simulink model "sltestRollRefTestExample"  (R2019a)
settings: Solver=FixedStepDiscrete  StartTime=0.0  StopTime=50  RelTol=1e-3
libraries: simulink x1, simulink_need_slupdate x1
settings Model: Creator=The MathWorks, Inc.  LastModifiedBy=sjayagop
settings DataIOCC: ReturnWorkspaceOutputs=off
settings DebuggingCC: PregeneratedLibrarySubsystemCodeDiagnostic=none  SFUnusedDataAndEventsDiag=none  ArithmeticOperatorsInVariantConditions=warning
settings SFSimCC: SimUseLocalCustomCode=off
settings RTWCC: RTWUseLocalCustomCode=off
settings CodeAppCC: StateflowObjectComments=on
settings ConfigComp: CovMetricSettings=dswe

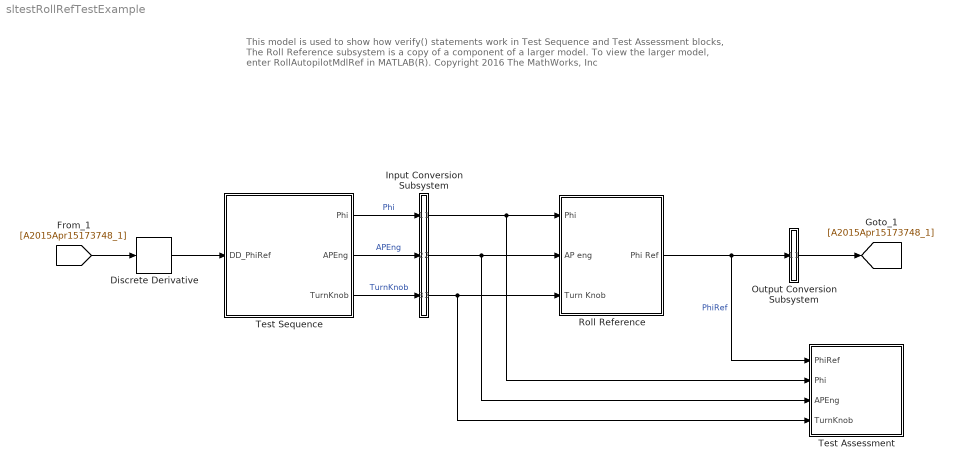
== system sltestRollRefTestExample ==
  note: This model is used to show how verify() statements work in Test Sequence and Test Assessment blocks,
      | The Roll Reference subsystem is a copy of a component of a larger model.
      | To view the larger model, enter RollAutopilotMdlRef in MATLAB(R).
      |
      | Copyright 2016 The MathWorks, Inc
  Discrete Derivative : simulink/Discrete/Discrete Derivative  gainval=1.0  ICPrevScaledInput=0.0  OutMin=[]  OutMax=[]  OutDataType=fixdt(1, 16)  OutScaling=2^-10  DoSatur=off
  Input Conversion Subsystem : Subsystem  Tag=_input_conv_ss_
  Output Conversion Subsystem : Subsystem  Tag=_output_conv_ss_
  Roll Reference : Subsystem  RequirementInfo={'other' 'RollAutopilotRequirements.txt' '?1.3 Roll Hold Reference' 'true' '1.3 Roll Hold Reference' '' } %GIDa_a6fe2b3a_fc40_48ad_979d_ac7ba21092bc  TreatAsAtomicUnit=on
      settings: RTWSystemCode=Inline
  Test Assessment : Test Sequence  TreatAsAtomicUnit=on
  Test Sequence : Test Sequence  RequirementInfo={'linktype_rmi_testmgr' 'AutopilotTestFile.mldatx' '635fd623-8d91-4a63-9a87-5e8aa5687fc0' 'true' 'Test Case Requirement 1.3 Test in AutopilotTestFile' '' } %GIDa_03a19a86_3761_446b_82d3_438f47eaa67c  TreatAsAtomicUnit=on
  wires:
  [A2015Apr15173748_1] -> Discrete Derivative/1
  Test Sequence/1(Phi) -> Input Conversion Subsystem/1(In_1)  "Phi"
  Test Sequence/2(APEng) -> Input Conversion Subsystem/2(In_2)  "APEng"
  Test Sequence/3(TurnKnob) -> Input Conversion Subsystem/3(In_3)  "TurnKnob"
  Input Conversion Subsystem/1(Out_1) -> Roll Reference/1(Phi), Test Assessment/2(Phi)
  Input Conversion Subsystem/2(Out_2) -> Roll Reference/2(AP eng), Test Assessment/3(APEng)
  Input Conversion Subsystem/3(Out_3) -> Roll Reference/3(Turn Knob), Test Assessment/4(TurnKnob)
  Roll Reference/1(Phi Ref) -> Test Assessment/1(PhiRef), Output Conversion Subsystem/1(In_1)  "PhiRef"
  Output Conversion Subsystem/1(Out_1) -> [A2015Apr15173748_1]
  Discrete Derivative/1 -> Test Sequence/1(DD_PhiRef)

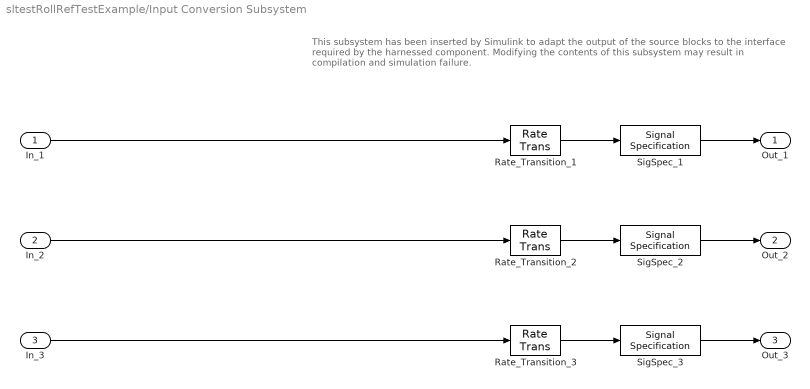
== system sltestRollRefTestExample/Input Conversion Subsystem ==
  note: This subsystem has been inserted by Simulink to adapt the output of the source blocks to the interface required by the harnessed component.
      |  Modifying the contents of this subsystem may result in compilation and simulation failure.
  In_1 : Inport
  In_2 : Inport  Port=2
  In_3 : Inport  Port=3
  Rate_Transition_1 : RateTransition  OutPortSampleTime=0.025
  Rate_Transition_2 : RateTransition  OutPortSampleTime=0.025
  Rate_Transition_3 : RateTransition  OutPortSampleTime=0.025
  SigSpec_1 : SignalSpecification  OutDataTypeStr=double  Dimensions=[1]  SampleTime=0.025
  SigSpec_2 : SignalSpecification  OutDataTypeStr=boolean  Dimensions=[1]  SampleTime=0.025
  SigSpec_3 : SignalSpecification  OutDataTypeStr=double  Dimensions=[1]  SampleTime=0.025
  Out_1 : Outport
  Out_2 : Outport  Port=2
  Out_3 : Outport  Port=3
  wires:
  In_1/1 -> Rate_Transition_1/1
  In_2/1 -> Rate_Transition_2/1
  In_3/1 -> Rate_Transition_3/1
  Rate_Transition_1/1 -> SigSpec_1/1
  Rate_Transition_2/1 -> SigSpec_2/1
  Rate_Transition_3/1 -> SigSpec_3/1
  SigSpec_1/1 -> Out_1/1
  SigSpec_2/1 -> Out_2/1
  SigSpec_3/1 -> Out_3/1

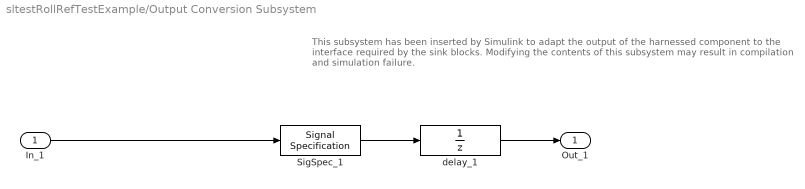
== system sltestRollRefTestExample/Output Conversion Subsystem ==
  note: This subsystem has been inserted by Simulink to adapt the output of the harnessed component to the interface required by the sink blocks.
      |  Modifying the contents of this subsystem may result in compilation and simulation failure.
  In_1 : Inport
  SigSpec_1 : SignalSpecification  OutDataTypeStr=double  Dimensions=[1]  SampleTime=0.025
  delay_1 : UnitDelay  SampleTime=-1  HasFrameUpgradeWarning=on
  Out_1 : Outport
  wires:
  delay_1/1 -> Out_1/1
  SigSpec_1/1 -> delay_1/1
  In_1/1 -> SigSpec_1/1

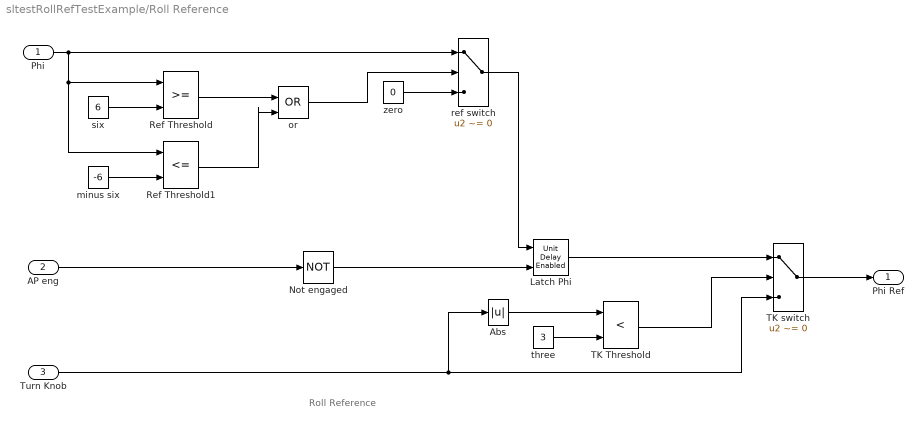
== system sltestRollRefTestExample/Roll Reference ==
  note: Roll Reference
  Phi : Inport  RequirementInfo={'other' 'RollAutopilotRequirements.txt' '?1.3 Roll Hold Reference' 'true' '1.3 Roll Hold Reference' '' } %GIDa_191cb6f5_9fbe_4640_9b65_3b39d8becb52
  AP eng : Inport  RequirementInfo={'other' 'RollAutopilotRequirements.txt' '?1.3 Roll Hold Reference' 'true' '1.3 Roll Hold Reference' '' } %GIDa_123acc0c_25f5_45e7_ac3a_1f2518b48f3f  Port=2
  Turn Knob : Inport  RequirementInfo={'other' 'RollAutopilotRequirements.txt' '?1.3 Roll Hold Reference' 'true' '1.3 Roll Hold Reference' '' } %GIDa_b6599344_476f_4c9f_9990_af58eba30b01  Port=3
  Abs : Abs  RequirementInfo={'other' 'RollAutopilotRequirements.txt' '?1.3 Roll Hold Reference' 'true' '1.3 Roll Hold Reference' '' } %GIDa_3ae1946e_a95c_4cb7_ad5c_447f76069b53
  Latch Phi : simulink_need_slupdate/Unit Delay Enabled  RequirementInfo={'other' 'RollAutopilotRequirements.txt' '?1.3 Roll Hold Reference' 'true' '1.3 Roll Hold Reference' '' } %GIDa_4d4d235f_0389_4d32_a678_f192d33a24f1  vinit=0.0  tsamp=1/40
      settings: SourceProductName=Simulink  SourceProductBaseCode=SL
  Not engaged : Logic  RequirementInfo={'other' 'RollAutopilotRequirements.txt' '?1.3 Roll Hold Reference' 'true' '1.3 Roll Hold Reference' '' } %GIDa_f773b49d_367f_448f_8750_15955fcab6a4  Operator=NOT  IconShape=distinctive  AllPortsSameDT=off  OutDataTypeStr=boolean
  Ref Threshold : RelationalOperator  RequirementInfo={'other' 'RollAutopilotRequirements.txt' '?1.3 Roll Hold Reference' 'true' '1.3 Roll Hold Reference' '' } %GIDa_215460f1_09d0_4074_847e_2cd07dedce05  OutDataTypeStr=boolean  RndMeth=Nearest  InputSameDT=on
  Ref Threshold1 : RelationalOperator  RequirementInfo={'other' 'RollAutopilotRequirements.txt' '?1.3 Roll Hold Reference' 'true' '1.3 Roll Hold Reference' '' } %GIDa_bbe88d87_da81_4bf6_a41e_c7cf823cfa2e  Operator=<=  OutDataTypeStr=boolean  RndMeth=Nearest  InputSameDT=on
  TK Threshold : RelationalOperator  RequirementInfo={'other' 'RollAutopilotRequirements.txt' '?1.3 Roll Hold Reference' 'true' '1.3 Roll Hold Reference' '' } %GIDa_315407ac_4ac8_4751_b85f_bc63ef605254  Operator=<  OutDataTypeStr=boolean  RndMeth=Nearest  InputSameDT=on
  TK switch : Switch  RequirementInfo={'other' 'RollAutopilotRequirements.txt' '?1.3 Roll Hold Reference' 'true' '1.3 Roll Hold Reference' '' } %GIDa_fe63e81b_e734_4e16_865c_d9a3984a5c48  Criteria=u2 ~= 0
  minus six : Constant  RequirementInfo={'other' 'RollAutopilotRequirements.txt' '?1.3 Roll Hold Reference' 'true' '1.3 Roll Hold Reference' '' } %GIDa_dc652bd8_503a_41e7_bbad_342aba540a4b  Value=-6
  or : Logic  RequirementInfo={'other' 'RollAutopilotRequirements.txt' '?1.3 Roll Hold Reference' 'true' '1.3 Roll Hold Reference' '' } %GIDa_a4e94f61_1fba_4385_a203_46c343f95573  Operator=OR  IconShape=distinctive  OutDataTypeStr=boolean
  ref switch : Switch  RequirementInfo={'other' 'RollAutopilotRequirements.txt' '?1.3 Roll Hold Reference' 'true' '1.3 Roll Hold Reference' '' } %GIDa_b10e5edf_5f89_41a5_89be_95c1d2d542e4  Criteria=u2 ~= 0
  six : Constant  RequirementInfo={'other' 'RollAutopilotRequirements.txt' '?1.3 Roll Hold Reference' 'true' '1.3 Roll Hold Reference' '' } %GIDa_d286ae6b_2de1_4987_9a0a_078f5969643a  Value=6
  three : Constant  RequirementInfo={'other' 'RollAutopilotRequirements.txt' '?1.3 Roll Hold Reference' 'true' '1.3 Roll Hold Reference' '' } %GIDa_0f242fd2_1100_4ff5_8b3c_b98deadb2dcf  Value=3  OutDataTypeStr=double
  zero : Constant  RequirementInfo={'other' 'RollAutopilotRequirements.txt' '?1.3 Roll Hold Reference' 'true' '1.3 Roll Hold Reference' '' } %GIDa_59393c31_3566_4647_b17b_08530a6ace5c  Value=0
  Phi Ref : Outport  RequirementInfo={'other' 'RollAutopilotRequirements.txt' '?1.3 Roll Hold Reference' 'true' '1.3 Roll Hold Reference' '' } %GIDa_c05d8fc8_23e5_4d44_a72f_87287db952d9
  wires:
  Not engaged/1 -> Latch Phi/2
  ref switch/1 -> Latch Phi/1
  Latch Phi/1 -> TK switch/1
  TK Threshold/1 -> TK switch/2
  Turn Knob/1 -> TK switch/3, Abs/1
  three/1 -> TK Threshold/2
  Abs/1 -> TK Threshold/1
  Phi/1 -> ref switch/1, Ref Threshold1/1, Ref Threshold/1
  AP eng/1 -> Not engaged/1
  TK switch/1 -> Phi Ref/1
  six/1 -> Ref Threshold/2
  zero/1 -> ref switch/3
  or/1 -> ref switch/2
  Ref Threshold/1 -> or/1
  Ref Threshold1/1 -> or/2
  minus six/1 -> Ref Threshold1/2

== stateflow chart sltestRollRefTestExample/Test Assessment ==
  settings: stateMachineType=SIMPLIFIED_MACHINE
  state GlobalAssessment
    state NormalRange
      verify((~(PhiRef < Phi) && ~(PhiRef > Phi)),'Simulink:verify_normal','PhiRef must equal Phi for normal operation')
    state BelowLowLimit
      verify((~(PhiRef < 0) && ~(PhiRef > 0)),'Simulink:verify_low','PhiRef must equal 0 for low angle operation')
    state ExceedPosLimit
      verify((~(PhiRef < 30) && ~(PhiRef > 30)),'Simulink:verify_high','PhiRef must equal 30 for high pos angle operation')
    state ExceedNegLimit
      verify((~(PhiRef < -30) && ~(PhiRef > 30)),'Simulink:verify_high','PhiRef must equal -30 for high neg angle operation')
    state TurnKnobAssessments
      state BelowLowTKLimit
        verify((~(PhiRef < 0) && ~(PhiRef > 0)),'Simulink:verifyTKLow','PhiRef must equal 0 for low TK operation')
      state NormalTKLimit
        verify((~(PhiRef < TurnKnob) && ~(PhiRef > TurnKnob)),'Simulink:verifyTKNormal','PhiRef must equal TurnKnob for normal TK operation')
      state Else2
      (default) -> (junction 102)
      TurnKnobAssessments -> (junction 102)
      (junction 102) -> (junction 103) [order 1] : [abs(Phi) < 3]
      (junction 103) -> BelowLowTKLimit [order 1] : [~in(BelowLowTKLimit)]
      (junction 102) -> (junction 113) [order 2]
      (junction 103) -> (junction 106) [order 2]
      (junction 113) -> (junction 114) [order 1] : [abs(Phi) >=3 && Phi <= 30]
      (junction 114) -> NormalTKLimit [order 1] : [~in(NormalTKLimit)]
      (junction 114) -> (junction 117) [order 2]
      (junction 120) -> (junction 121)
      (junction 121) -> Else2 [order 1] : [~in(Else2)]
      (junction 121) -> (junction 124) [order 2]
      (junction 113) -> (junction 120) [order 2]
    state Else1
    GlobalAssessment -> (junction 22)
    (default) -> (junction 22)
    (junction 22) -> (junction 23) [order 1] : [(abs(Phi) >= 6 && Phi <= 30) && APEng == true && TurnKnob == false]
    (junction 23) -> NormalRange [order 1] : [~in(NormalRange)]
    (junction 22) -> (junction 46) [order 2]
    (junction 23) -> (junction 26) [order 2]
    (junction 46) -> (junction 47) [order 1] : [abs(Phi) < 6 && APEng == true && TurnKnob == false]
    (junction 47) -> BelowLowLimit [order 1] : [~in(BelowLowLimit)]
    (junction 46) -> (junction 73) [order 2]
    (junction 47) -> (junction 50) [order 2]
    (junction 73) -> (junction 74) [order 1] : [Phi > 30 && APEng == true && TurnKnob == false]
    (junction 74) -> ExceedPosLimit [order 1] : [~in(ExceedPosLimit)]
    (junction 73) -> (junction 84) [order 2]
    (junction 74) -> (junction 77) [order 2]
    (junction 84) -> (junction 85) [order 1] : [Phi < -30 && APEng == true && TurnKnob == false]
    (junction 85) -> ExceedNegLimit [order 1] : [~in(ExceedNegLimit)]
    (junction 84) -> (junction 62) [order 2]
    (junction 85) -> (junction 88) [order 2]
    (junction 62) -> (junction 63) [order 1] : [APEng == true && TurnKnob == true]
    (junction 63) -> TurnKnobAssessments [order 1] : [~in(TurnKnobAssessments)]
    (junction 62) -> (junction 31) [order 2]
    (junction 63) -> (junction 66) [order 2]
    (junction 31) -> (junction 32)
    (junction 32) -> Else1 [order 1] : [~in(Else1)]
    (junction 32) -> (junction 35) [order 2]
  (default) -> GlobalAssessment
  data: PhiRef input; Phi input; APEng input; TurnKnob input

== stateflow chart sltestRollRefTestExample/Test Sequence ==
  settings: stateMachineType=SIMPLIFIED_MACHINE
  state InitializeTest
    Phi = 0;
    APEng = false;
    TurnKnob = 0;
    % Initializes test sequence outputs
  state AttitudeLevels
    TurnKnob = 0;
    EndTest = 0;
    % Tests correct PhiRef for several attitudes with 0 turn knob
    state APEngage_LowRoll
      % Tests low attitude
      state SetLowPhi
        Phi = 4;
        APEng = false;
      state EngageAP_Low
        APEng = true;
      (default) -> SetLowPhi
      SetLowPhi -> EngageAP_Low : [true]
    state APEngage_MedRoll
      % Tests medium attitude
      state SetMedPhi
        Phi = 11.5;
        APEng = false;
      state EngageAP_Med
        APEng = true;
      (default) -> SetMedPhi
      SetMedPhi -> EngageAP_Med : [true]
    state APEngage_HighRoll
      % Tests high attitude
      state SetHighPhi
        Phi = 30.6;
        APEng = false;
      state EngageAP_High
        APEng = true;
      (default) -> SetHighPhi
      SetHighPhi -> EngageAP_High : [true]
    state APEngagement_End
      EndTest = 1;
    (default) -> APEngage_LowRoll
    APEngage_LowRoll -> APEngage_MedRoll : [duration(DD_PhiRef == 0,sec) >= DurationLimit
        |
        | % transitions when the discrete derivative of PhiRef
        | % is equal to 0 for a certain time limit. This means the
        | % signal is not changing.
        | ]
    APEngage_MedRoll -> APEngage_HighRoll : [duration(DD_PhiRef == 0,sec) >= DurationLimit]
    APEngage_HighRoll -> APEngagement_End : [duration(DD_PhiRef == 0,sec) >= DurationLimit]
  state TurnKnobLevels
    EndTest = 0;
    Phi = 0;
    % Tests correct PhiRef for several knob settings with 0 attitude
    state InitializeAPKnob
      TurnKnob = 0;
      APEng = false;
    state TurnKnobLow
      % Tests low knob setting
      state SetKnobLow
        TurnKnob = 2;
        APEng = false;
      state EngageAP_KnobLow
        APEng = true;
      SetKnobLow -> EngageAP_KnobLow : [true]
      (default) -> SetKnobLow
    state TurnKnobHigh
      % Tests high knob settings
      state SetKnobHigh
        TurnKnob = 17.3;
        APEng = false;
      state EngageAP_KnobHigh
        APEng = true;
      SetKnobHigh -> EngageAP_KnobHigh : [true]
      (default) -> SetKnobHigh
    state KnobTestEnd
      EndTest = 1;
    (default) -> InitializeAPKnob
    InitializeAPKnob -> TurnKnobLow : [true]
    TurnKnobLow -> TurnKnobHigh : [duration(DD_PhiRef == 0,sec) >= DurationLimit]
    TurnKnobHigh -> KnobTestEnd : [duration(DD_PhiRef == 0,sec) >= DurationLimit]
  state TurnKnobAndAttitude
    % Tests correct PhiRef for turn knob setting and attitude
    state InitializeTKandPhi
      APEng = false;
    state SetKnobAndPhi
      Phi = 4.5;
      TurnKnob = 5.1;
    state EngageAP
      APEng = true;
    InitializeTKandPhi -> SetKnobAndPhi : [true]
    (default) -> InitializeTKandPhi
    SetKnobAndPhi -> EngageAP : [true]
  state Stop
    APEng = false;
    Phi = 0;
    TurnKnob = 0;
  (default) -> InitializeTest
  InitializeTest -> AttitudeLevels : [true
      | ]
  AttitudeLevels -> TurnKnobLevels : [EndTest == 1]
  TurnKnobLevels -> TurnKnobAndAttitude : [EndTest == 1]
  TurnKnobAndAttitude -> Stop : [duration(DD_PhiRef == 0,sec) >= DurationLimit]
  data: Phi output double size=[1]; APEng output boolean size=[1]; TurnKnob output double size=[1]; DD_PhiRef input; DurationLimit constant double =5; EndTest local =0
